simulink model "idm"  (R2013a)
settings: Solver=ode45  StartTime=0.0  StopTime=10.0  RelTol=1e-3
libraries: powerlib x6
settings Model: Creator=User  LastModifiedBy=User

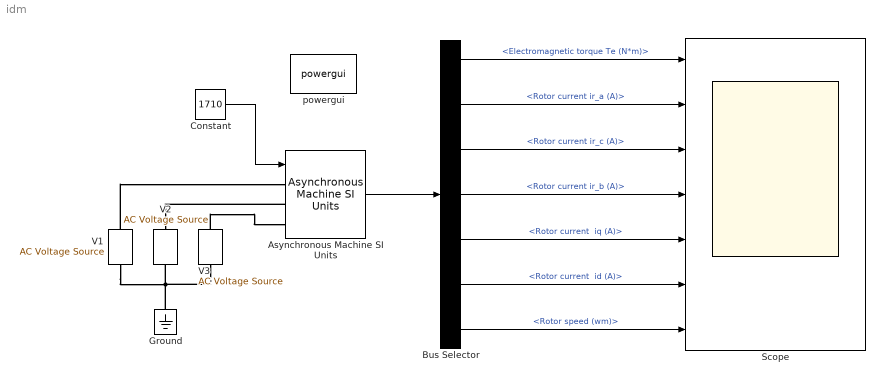
== system idm ==
  Asynchronous Machine SI Units : powerlib/Machines/Asynchronous Machine SI Units  PresetModel=No  MechanicalLoad=Speed w  ShowDetailedParameters=on  RotorType=Squirrel-cage  ReferenceFrame=Rotor  NominalParameters=[ 3*746, 220, 50 ]  Stator=[ 0.435 0.0024]  Rotor=[ 0.8160 0.0024]  Cage1=[ 0.022 0.226/377]  Cage2=[ 0.022 0.226/377]  Lm=0.08317  Mechanical="[ 0.0890 0  2 ]"  PolePairs=2  InitialConditions=[1 0 0 0 0 0 0 0]  Units=SI  LoadFlowParameters=1492000  SimulateSaturation=off  Saturation=[14.03593122, 27.81365428, 53.79336849, 72.68890987, 97.98006896, 148.6815601, 215.7428561, 302.9841135, 420.4778367 ; 230, 322, 414, 460, 506, 552, 598, 644, 690]  TsPowergui=0  TsBlock=-1  IterativeModel=Trapezoidal non iterative  Pmec=0
  Bus Selector : BusSelector  OutputSignals="Mechanical.Electromagnetic torque Te (N*m),Rotor measurements.Rotor current ir_a (A),Rotor measurements.Rotor current ir_c (A),Rotor measurements.Rotor current ir_b (A),Rotor measurements.Rotor current  iq (A),Rotor measurements.Rotor current  id (A),Mechanical.Rotor speed (wm)"
  Constant : Constant  Value=1710
  Ground : powerlib/Elements/Ground  LConnTagsString=a
  Scope : Scope  NumInputPorts=7
      settings: TimeRange=10  YMin=-80~-200~-200~-200~-200~-200~1709  YMax=0~200~200~200~200~200~1711  SampleTime=10
  V1 : powerlib/Electrical Sources/AC Voltage Source  Amplitude=311.126  Phase=0  Frequency=50  SampleTime=0  Measurements=None
  V2 : powerlib/Electrical Sources/AC Voltage Source  Amplitude=311.126  Phase=120  Frequency=50  SampleTime=0  Measurements=None
  V3 : powerlib/Electrical Sources/AC Voltage Source  Amplitude=311.126  Phase=240  Frequency=50  SampleTime=0  Measurements=None
  powergui : powerlib/powergui  Priority=1  SimulationMode=Continuous  SolverType=Tustin  SampleTime=50e-6  frequency=60  SPID=off  DisableSnubberDevices=off  DisableRonSwitches=off  DisableVfSwitches=off  SwTol=0  Interpol=off  DisplayEquations=off  frequencyindice=50  Pbase=100e6  ErrMax=1e-4  Iterations=50  UnitsV=kV  UnitsW=MW  FunctionMessages=off  echomessages=off  HookPort=off  EnableUseOfTLC=off  x0status=blocks  RestoreLinks=warning  ResistiveCurrentMeasurement=off  Frange=[0:2:500]  Ylog=off  Xlog=on  ShowGrid=off  save=off  variable=ZData  ZoomFFT=off  StartTime=0.0  cycles=1  DisplayStyle=1  fundamental=60  FreqAxis=off  MaxFrequency=1000  frequencyindicesteady=1  RmsSteady=1  display=off  Ts=0  methode=off
  wires:
  Asynchronous Machine SI Units/1 -> Bus Selector/1
  Bus Selector/1 -> Scope/1  "<Electromagnetic torque Te (N*m)>"
  Constant/1 -> Asynchronous Machine SI Units/1
  Bus Selector/4 -> Scope/4  "<Rotor current ir_b (A)>"
  Bus Selector/5 -> Scope/5  "<Rotor current  iq (A)>"
  Bus Selector/3 -> Scope/3  "<Rotor current ir_c (A)>"
  Bus Selector/6 -> Scope/6  "<Rotor current  id (A)>"
  Bus Selector/2 -> Scope/2  "<Rotor current ir_a (A)>"
  Bus Selector/7 -> Scope/7  "<Rotor speed (wm)>"
  connections:
  V1/RConn1 -- Asynchronous Machine SI Units/LConn1
  Asynchronous Machine SI Units/LConn2 -- V2/RConn1
  V1/LConn1 -- Ground/LConn1 -- V3/LConn1 -- V2/LConn1
  V3/RConn1 -- Asynchronous Machine SI Units/LConn3
